simulink model "lab2_simulink"  (R2024b)
settings: Solver=VariableStepAuto  StartTime=0.0  StopTime=10000  RelTol=1e-3
settings Model: Creator=stefa  LastModifiedBy=stefa

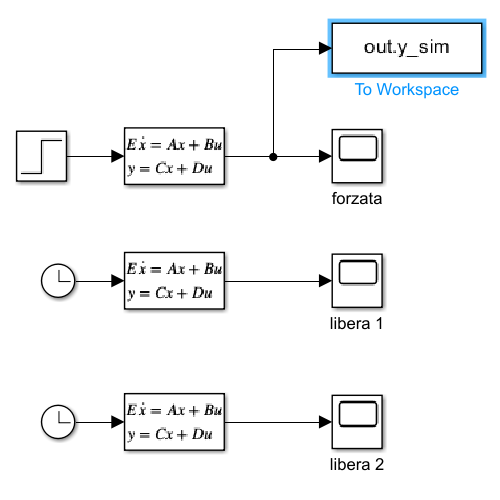
[thumbnail: Simulink's stored preview of the top-level diagram]
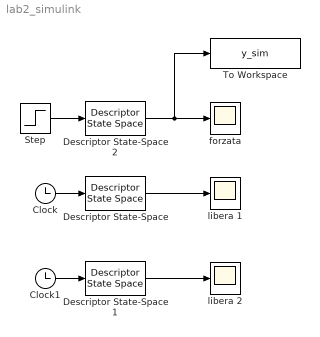
== system lab2_simulink ==
  Clock : Clock
  Clock1 : Clock
  Descriptor State-Space : DescriptorStateSpace  E=eye(3)  A=[0 -1 5; 0 0 3; 0 0 -2]  B=[0 0 0]'  C=[0 0 5]  D=0  InitialCondition=[1 5 0]'
  Descriptor State-Space1 : DescriptorStateSpace  E=eye(3)  A=[0 -1 5; 0 0 3; 0 0 -2]  B=[0 0 0]'  C=[0 0 5]  D=0  InitialCondition=[0 0 3]'
  Descriptor State-Space2 : DescriptorStateSpace  E=eye(3)  A=[0 -1 5; 0 0 3; 0 0 -2]  B=[1 1 1]'  C=[0 0 5]  D=0  InitialCondition=[0 0 0]'
  Step : Step  Time=0  After=9  SampleTime=0
  To Workspace : ToWorkspace  VariableName=y_sim  SaveFormat=Structure With Time  SampleTime=-1
  forzata : Scope
  libera 1 : Scope
  libera 2 : Scope
  wires:
  Clock/1 -> Descriptor State-Space/1
  Descriptor State-Space/1 -> libera 1/1
  Descriptor State-Space1/1 -> libera 2/1
  Clock1/1 -> Descriptor State-Space1/1
  Descriptor State-Space2/1 -> To Workspace/1, forzata/1
  Step/1 -> Descriptor State-Space2/1
